simulink model "Kubon_lab5_sim"  (R2020b)
settings: Solver=VariableStepAuto  StartTime=0.0  StopTime=10.0  MaxStep=0.01  RelTol=1e-3
values from neighbouring files (symbols this model uses):
  b = Cv1*Cv2    (= 308700000)    [Kubon_lab13.m]    (also in Kubon_lab4.m = 8; Kubon_lab5.m = 2*ksi(i)*w(i); Kubon_poprawa_lab5.m = 2*e(i)*w(i))
  c = (Cv1*a_1+Cv1*ks2+Cv1*k0+Cv2*a_1+Cv2*ks1+Cv2*k0)    (= 68544000)    [Kubon_lab13.m]    (also in Kubon_lab5.m = w(i)*w(i); Kubon_poprawa_lab5.m = w(i)^2)
  d0 = 1    [Kubon_lab5.m]    (also in Kubon_poprawa_lab5.m)
  t0 = 50.0    (= 50)    [Kubon_lab10.m]    (also in Kubon_lab4.m = 5; Kubon_lab5.m = 0; Kubon_lab6.m = 5; Kubon_lab6_test.m = 0)
  u0 = 3    [Kubon_lab4.m]    (also in Kubon_lab5.m = 0; Kubon_poprawa_lab5.m = 0)
  x0 = 0    [Kubon_lab4.m]    (also in Kubon_lab5.m; Kubon_lab8.m = [h10,h20])
  x10 = 0    [Kubon_lab5.m]    (also in Kubon_poprawa_lab5.m)
settings Model: Creator=Weronika  LastModifiedBy=pkubo
settings DataIOCC: SaveFormat=Array  ReturnWorkspaceOutputs=off

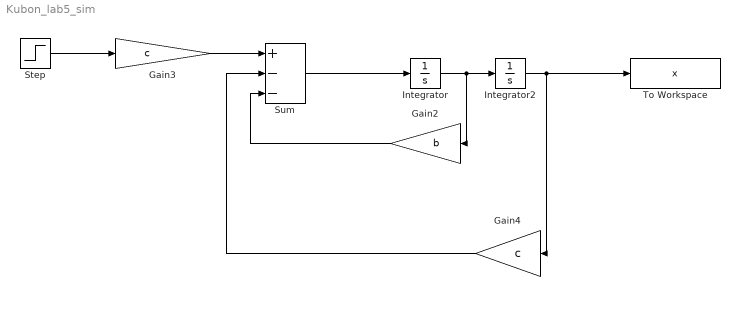
== system Kubon_lab5_sim ==
  Gain2 : Gain  Gain=b
  Gain3 : Gain  Gain=c
  Gain4 : Gain  Gain=c
  Integrator : Integrator  InitialCondition=x10
  Integrator2 : Integrator  InitialCondition=x0
  Step : Step  Time=t0  Before=u0  After=u0+d0  SampleTime=0
  Sum : Sum  Inputs=+--
  To Workspace : ToWorkspace  VariableName=x  SampleTime=-1
  wires:
  Sum/1 -> Integrator/1
  Integrator/1 -> Integrator2/1, Gain2/1
  Integrator2/1 -> Gain4/1, To Workspace/1
  Gain2/1 -> Sum/3
  Gain4/1 -> Sum/2
  Gain3/1 -> Sum/1
  Step/1 -> Gain3/1
